simulink model "gm_sampleModel1912_4_sub"  (R2023a)
settings: Solver=VariableStepAuto  StartTime=0.0  StopTime=10.0  RelTol=1e-3
libraries: simulink x5
settings Model: Creator=user1  LastModifiedBy=user1
settings OptimizationCC: BlockReduction=off  ConditionallyExecuteInputs=off
settings DebuggingCC: InheritedTsInSrcMsg=none

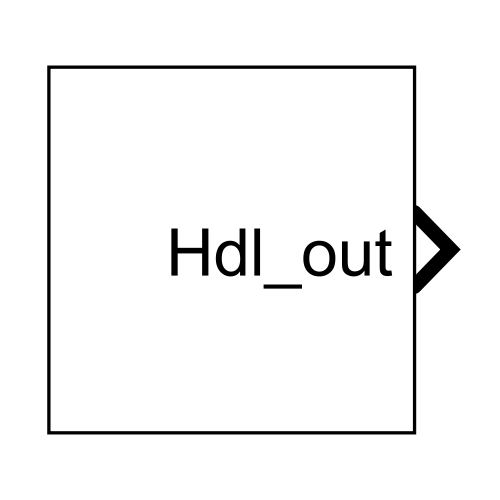
[thumbnail: Simulink's stored preview of the top-level diagram]
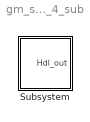
== system gm_sampleModel1912_4_sub ==
  Subsystem : Subsystem

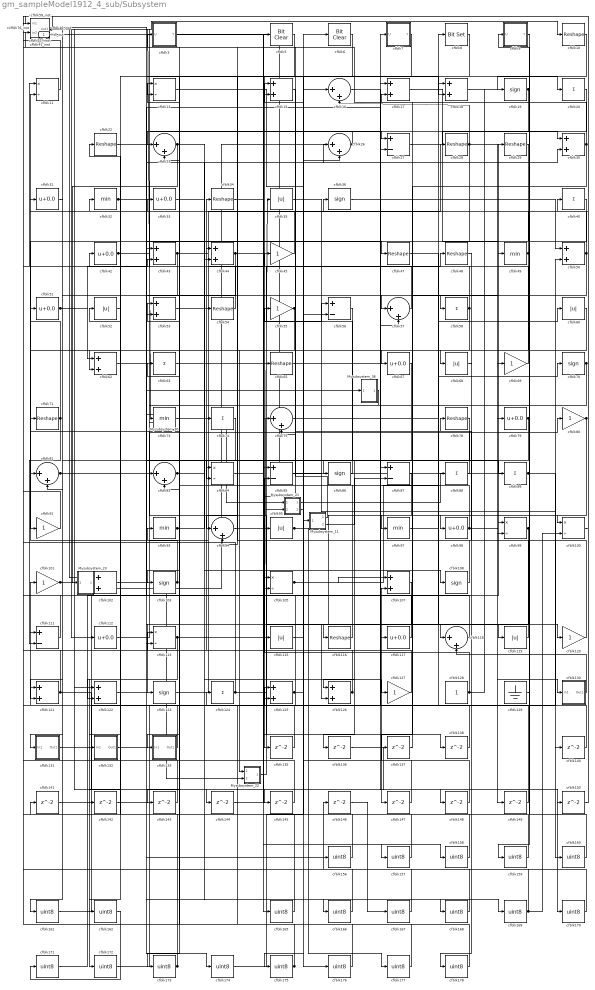
== system gm_sampleModel1912_4_sub/Subsystem ==
  Mysubsystem_11 : Subsystem
  Mysubsystem_21 : Subsystem
  Mysubsystem_22 : Subsystem
  Mysubsystem_23 : Subsystem
  Mysubsystem_30 : Subsystem
  Mysubsystem_36 : Subsystem
  cfblk{10,22,28..29,34,47..48,54,65,71,78,116} (12 alike) : Reshape
  cfblk{11,13,84,99..100,105,113} (7 alike) : Product  Inputs=*/  OutDataTypeStr=uint8  RndMeth=Zero  SaturateOnIntegerOverflow=on
  cfblk{45,55,69,80,91,101,120,127} (8 alike) : Gain  OutDataTypeStr=uint8
  cfblk{15,17..18,30,43..44,50,53,62,102,107,121..122,125..126} (15 alike) : Sum  OutDataTypeStr=uint8
  cfblk{19,36,70,86,103,108,123} (7 alike) : Signum
  cfblk106_inst : Subsystem
  cfblk{27,56,85,87,111} (5 alike) : Sum  Inputs=+-  OutDataTypeStr=uint8
  cfblk{31,33,42,51,67,79,98,112,117} (9 alike) : Bias  Bias=0.0  SaturateOnIntegerOverflow=off
  cfblk114_inst : Subsystem
  cfblk{35,52,60,68,95,115,119} (7 alike) : Abs  OutDataTypeStr=uint8  SaturateOnIntegerOverflow=off
  cfblk{16,23,26,57,75,81,83,94,118} (9 alike) : Sum  Inputs=|++  OutDataTypeStr=uint8
  cfblk{20,40,58,63,74,88..89,124} (8 alike) : Sum  Inputs=+  OutDataTypeStr=uint8
  cfblk128 : Constant  OutDataTypeStr=uint8  SampleTime=-1
  cfblk129 : Ground
  cfblk12_inst : Subsystem
  cfblk130 : Subsystem
  cfblk131 : Subsystem
  cfblk132 : Subsystem
  cfblk133 : Subsystem
  cfblk{135..138,140..150} (15 alike) : Delay  SampleTime=1
  cfblk14_inst : Subsystem
  cfblk{156..162,165..178} (21 alike) : DataTypeConversion  OutDataTypeStr=uint8  SaturateOnIntegerOverflow=off  RndMeth=Floor
  cfblk21_inst : Subsystem
  cfblk24_inst : Subsystem
  cfblk3 : Subsystem  mask(Detect Rise Positive){vinit=double(0), InputProcessing=Elements as channels (sample based), OutDataTypeStr=uint8}
      mask prompts: vinit "Simulink:masks:InitialCondition_MP"; InputProcessing "Simulink:masks:InputProcessing_MP"; OutDataTypeStr "Simulink:masks:OutputDataType_MP"
      mask help: Simulink:masks:DetectRisePositive_MD
      mask init:
      | InputProcessing = 'Elements as channels (sample based)';
      | OutDataTypeStr = 'uint8';
      | vinit = double(0);
      mask TypeOptions InputProcessing: Simulink:masks:ColumnsAsChannelsFrameBased | Simulink:masks:ElementsAsChannelsSampleBased
      mask TypeOptions OutDataTypeStr: Simulink:masks:uint8 | Simulink:masks:boolean
      mask Display: fprintf('U > 0\n&  NOT\nU/z > 0')
  cfblk{32,49,73,93,97} (5 alike) : MinMax  OutDataTypeStr=uint8
  cfblk37_inst : Subsystem
  cfblk38_inst : Subsystem
  cfblk4 : Constant  Value=0  OutDataTypeStr=uint8  SampleTime=1
  cfblk41_inst : Subsystem
  cfblk46_inst : Subsystem
  cfblk5 : simulink/Logic and Bit Operations/Bit Clear  iBit=0
      settings: LibrarySourceBlock=|
      | hdlsllib/Logic and Bit
      | Operations/Bit Clear
  cfblk59_inst : Subsystem
  cfblk6 : simulink/Logic and Bit Operations/Bit Clear  iBit=0
      settings: LibrarySourceBlock=|
      | hdlsllib/Logic and Bit
      | Operations/Bit Clear
  cfblk7 : Subsystem  mask(Detect Fall Nonpositive){vinit=double(0), InputProcessing=Elements as channels (sample based), OutDataTypeStr=uint8}
      mask prompts: vinit "Simulink:masks:InitialCondition_MP"; InputProcessing "Simulink:masks:InputProcessing_MP"; OutDataTypeStr "Simulink:masks:OutputDataType_MP"
      mask help: Simulink:masks:DetectFallNonpositive_MD
      mask init:
      | InputProcessing = 'Elements as channels (sample based)';
      | OutDataTypeStr = 'uint8';
      | vinit = double(0);
      mask TypeOptions InputProcessing: Simulink:masks:ColumnsAsChannelsFrameBased | Simulink:masks:ElementsAsChannelsSampleBased
      mask TypeOptions OutDataTypeStr: Simulink:masks:uint8 | Simulink:masks:boolean
      mask Display: fprintf('U <= 0\n&  NOT\nU/z <= 0')
  cfblk76_inst : Subsystem
  cfblk8 : simulink/Logic and Bit Operations/Bit Set  iBit=0
      settings: LibrarySourceBlock=|
      | hdlsllib/Logic and Bit
      | Operations/Bit Set
  cfblk9 : Subsystem  mask(Detect Fall Nonpositive){vinit=double(0), InputProcessing=Elements as channels (sample based), OutDataTypeStr=uint8}
      mask prompts: vinit "Simulink:masks:InitialCondition_MP"; InputProcessing "Simulink:masks:InputProcessing_MP"; OutDataTypeStr "Simulink:masks:OutputDataType_MP"
      mask help: Simulink:masks:DetectFallNonpositive_MD
      mask init:
      | InputProcessing = 'Elements as channels (sample based)';
      | OutDataTypeStr = 'uint8';
      | vinit = double(0);
      mask TypeOptions InputProcessing: Simulink:masks:ColumnsAsChannelsFrameBased | Simulink:masks:ElementsAsChannelsSampleBased
      mask TypeOptions OutDataTypeStr: Simulink:masks:uint8 | Simulink:masks:boolean
      mask Display: fprintf('U <= 0\n&  NOT\nU/z <= 0')
  cfblk92_inst : Subsystem
  Hdl_out : Outport  OutDataTypeStr=uint8  SampleTime=1
  wires:
  Mysubsystem_11/1(Out1) -> cfblk46_inst/2(in2)
  Mysubsystem_11/2(Out2) -> cfblk87/2
  Mysubsystem_21/1(Out1) -> cfblk88/1
  Mysubsystem_21/2(Out2) -> Mysubsystem_11/1(In1)
  Mysubsystem_22/1(Out1) -> Mysubsystem_21/2(In2)
  Mysubsystem_23/1(Out1) -> Mysubsystem_22/2(In2)
  Mysubsystem_30/1(Out1) -> Mysubsystem_21/1(In1)
  Mysubsystem_36/1(Out1) -> Mysubsystem_30/2(In2)
  cfblk10/1 -> cfblk135/1
  cfblk100/1 -> cfblk37_inst/1(in1)
  cfblk101/1 -> cfblk145/1, cfblk144/1
  cfblk102/1 -> cfblk80/1
  cfblk103/1 -> cfblk11/2, cfblk93/1
  cfblk105/1 -> cfblk18/1, cfblk107/1
  cfblk106_inst/1(out1) -> cfblk119/1
  cfblk107/1 -> cfblk123/1
  cfblk108/1 -> cfblk24_inst/1(in1)
  cfblk11/1 -> cfblk38_inst/1(in1)
  cfblk111/1 -> cfblk12_inst/1(in1)
  cfblk112/1 -> cfblk36/1
  cfblk113/1 -> cfblk35/1, cfblk172/1
  cfblk114_inst/1(out1) -> cfblk106_inst/1(in1), cfblk147/1
  cfblk115/1 -> cfblk56/2
  cfblk116/1 -> cfblk114_inst/1(in1)
  cfblk117/1 -> cfblk21_inst/1(in1)
  cfblk118/1 -> cfblk21_inst/2(in2)
  cfblk119/1 -> cfblk78/1
  cfblk12_inst/1(out1) -> cfblk27/1, cfblk73/1
  cfblk120/1 -> cfblk3/1(U)
  cfblk121/1 -> cfblk38_inst/2(in2), cfblk29/1, cfblk148/1
  cfblk122/1 -> cfblk174/1
  cfblk123/1 -> cfblk45/1
  cfblk124/1 -> cfblk48/1, cfblk37_inst/2(in2)
  cfblk125/1 -> cfblk26/2, cfblk16/1
  cfblk126/1 -> cfblk34/1, cfblk101/1
  cfblk127/1 -> cfblk52/1
  cfblk128/1 -> cfblk85/2, cfblk19/1
  cfblk129/1 -> cfblk49/1
  cfblk13/1 -> cfblk176/1
  cfblk130/1(Out1) -> cfblk118/2
  cfblk131/1(Out1) -> cfblk7/1(U)
  cfblk132/1(Out1) -> cfblk125/1
  cfblk133/1(Out1) -> cfblk111/1
  cfblk135/1 -> cfblk92_inst/1(in1)
  cfblk136/1 -> cfblk170/1
  cfblk137/1 -> cfblk17/2
  cfblk138/1 -> cfblk83/2
  cfblk14_inst/1(out1) -> cfblk85/1, cfblk122/1
  cfblk140/1 -> cfblk99/1
  cfblk141/1 -> cfblk50/2
  cfblk142/1 -> cfblk57/2
  cfblk143/1 -> cfblk59_inst/2(in2)
  cfblk144/1 -> cfblk56/1
  cfblk145/1 -> cfblk12_inst/2(in2)
  cfblk146/1 -> cfblk167/1
  cfblk147/1 -> cfblk15/1
  cfblk148/1 -> cfblk107/2
  cfblk149/1 -> cfblk105/1
  cfblk15/1 -> cfblk95/1
  cfblk150/1 -> cfblk40/1
  cfblk156/1 -> cfblk14_inst/2(in2)
  cfblk157/1 -> cfblk41_inst/1(in1)
  cfblk158/1 -> cfblk41_inst/2(in2)
  cfblk159/1 -> cfblk42/1
  cfblk16/1 -> cfblk87/1
  cfblk160/1 -> cfblk9/1(U)
  cfblk161/1 -> cfblk5/1
  cfblk162/1 -> cfblk171/1
  cfblk165/1 -> cfblk46_inst/1(in1)
  cfblk166/1 -> cfblk63/1
  cfblk167/1 -> cfblk76_inst/1(in1)
  cfblk168/1 -> cfblk146/1
  cfblk169/1 -> cfblk59_inst/1(in1), cfblk100/2
  cfblk17/1 -> cfblk69/1
  cfblk170/1 -> cfblk53/1
  cfblk171/1 -> cfblk53/2
  cfblk172/1 -> cfblk8/1
  cfblk173/1 -> cfblk106_inst/2(in2), cfblk141/1
  cfblk174/1 -> cfblk6/1
  cfblk175/1 -> cfblk113/1, cfblk124/1
  cfblk176/1 -> cfblk14_inst/1(in1)
  cfblk177/1 -> cfblk13/1
  cfblk178/1 -> cfblk13/2
  cfblk18/1 -> cfblk20/1
  cfblk19/1 -> cfblk27/2, cfblk23/2
  cfblk20/1 -> cfblk84/2
  cfblk21_inst/1(out1) -> cfblk18/2
  cfblk22/1 -> cfblk47/1
  cfblk23/1 -> cfblk54/1, Mysubsystem_23/1(In1)
  cfblk24_inst/1(out1) -> cfblk166/1
  cfblk26/1 -> cfblk23/1, cfblk102/2
  cfblk27/1 -> cfblk30/1
  cfblk28/1 -> cfblk79/1, cfblk75/2, cfblk16/2
  cfblk29/1 -> cfblk91/1
  cfblk3/1(Y) -> cfblk157/1
  cfblk30/1 -> cfblk24_inst/2(in2), cfblk137/1
  cfblk31/1 -> cfblk131/1(In1)
  cfblk32/1 -> cfblk149/1, cfblk74/1
  cfblk33/1 -> cfblk58/1
  cfblk34/1 -> cfblk168/1
  cfblk35/1 -> cfblk140/1
  cfblk36/1 -> cfblk50/1
  cfblk37_inst/1(out1) -> Mysubsystem_30/1(In1)
  cfblk38_inst/1(out1) -> cfblk102/1
  cfblk4/1 -> cfblk57/1
  cfblk40/1 -> cfblk67/1
  cfblk41_inst/1(out1) -> cfblk156/1
  cfblk42/1 -> cfblk83/1, cfblk75/1
  cfblk43/1 -> cfblk28/1, cfblk122/2
  cfblk44/1 -> cfblk62/2, cfblk161/1, cfblk158/1
  cfblk45/1 -> cfblk32/1
  cfblk46_inst/1(out1) -> cfblk86/1
  cfblk47/1 -> cfblk120/1
  cfblk48/1 -> cfblk118/1
  cfblk49/1 -> cfblk31/1, cfblk178/1
  cfblk5/1 -> cfblk162/1
  cfblk50/1 -> cfblk15/2, cfblk97/1
  cfblk51/1 -> cfblk62/1, cfblk43/2
  cfblk52/1 -> cfblk142/1
  cfblk53/1 -> cfblk169/1
  cfblk54/1 -> cfblk11/1
  cfblk55/1 -> cfblk94/2, cfblk143/1
  cfblk56/1 -> cfblk132/1(In1)
  cfblk57/1 -> cfblk22/1
  cfblk58/1 -> cfblk81/1, cfblk44/1, Mysubsystem_22/1(In1)
  cfblk59_inst/1(out1) -> cfblk112/1
  cfblk6/1 -> cfblk175/1
  cfblk60/1 -> cfblk68/1
  cfblk62/1 -> Mysubsystem_36/1(In1)
  cfblk63/1 -> cfblk165/1
  cfblk65/1 -> cfblk150/1
  cfblk67/1 -> cfblk103/1
  cfblk68/1 -> cfblk98/1
  cfblk69/1 -> cfblk92_inst/2(in2)
  cfblk7/1(Y) -> cfblk84/1
  cfblk70/1 -> cfblk99/2, cfblk105/2
  cfblk71/1 -> cfblk51/1, cfblk111/2
  cfblk73/1 -> cfblk115/1
  cfblk74/1 -> cfblk121/2
  cfblk75/1 -> cfblk70/1
  cfblk76_inst/1(out1) -> cfblk81/2, cfblk89/1
  cfblk78/1 -> cfblk94/1
  cfblk79/1 -> cfblk126/1, cfblk121/1, cfblk116/1
  cfblk8/1 -> cfblk173/1
  cfblk80/1 -> cfblk126/2, cfblk100/1
  cfblk81/1 -> cfblk26/1, cfblk17/1
  cfblk83/1 -> cfblk33/1, cfblk30/2, cfblk108/1
  cfblk84/1 -> cfblk138/1
  cfblk85/1 -> cfblk117/1
  cfblk86/1 -> cfblk55/1
  cfblk87/1 -> cfblk136/1
  cfblk88/1 -> cfblk76_inst/2(in2)
  cfblk89/1 -> cfblk160/1, Hdl_out/1
  cfblk9/1(Y) -> cfblk159/1
  cfblk91/1 -> cfblk114_inst/2(in2)
  cfblk92_inst/1(out1) -> cfblk44/2, cfblk10/1
  cfblk93/1 -> cfblk65/1, cfblk125/2
  cfblk94/1 -> cfblk127/1
  cfblk95/1 -> cfblk43/1, cfblk177/1
  cfblk97/1 -> cfblk60/1
  cfblk98/1 -> cfblk71/1, cfblk130/1(In1)
  cfblk99/1 -> cfblk113/2, cfblk133/1(In1)

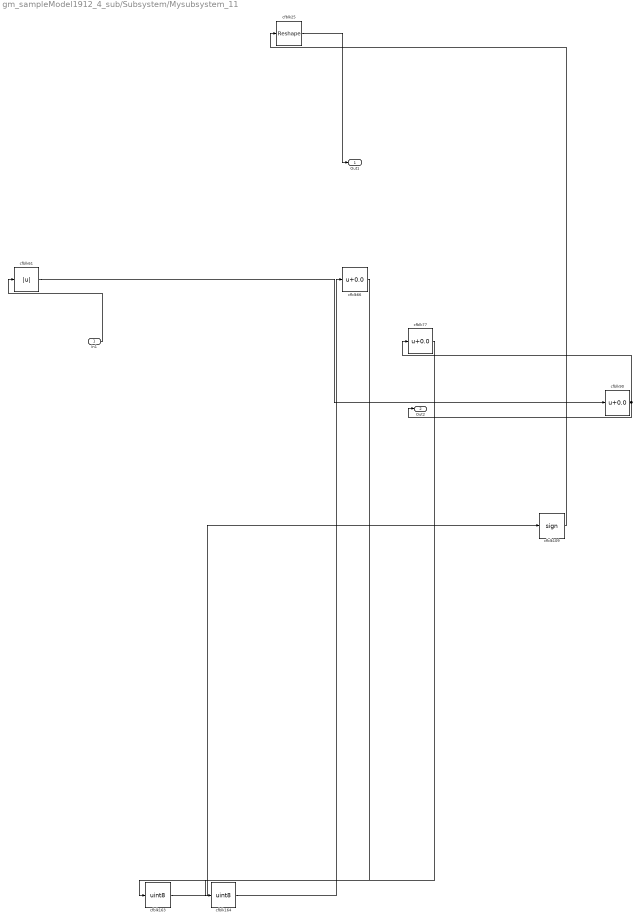
== system gm_sampleModel1912_4_sub/Subsystem/Mysubsystem_11 ==
  In1 : Inport  OutDataTypeStr=fixdt(0, 8, 7)  PortDimensions=1  SampleTime=1
  cfblk109 : Signum
  cfblk163 : DataTypeConversion  OutDataTypeStr=uint8  SaturateOnIntegerOverflow=off  RndMeth=Floor
  cfblk164 : DataTypeConversion  OutDataTypeStr=uint8  SaturateOnIntegerOverflow=off  RndMeth=Floor
  cfblk25 : Reshape
  cfblk61 : Abs  SaturateOnIntegerOverflow=off
  cfblk66 : Bias  Bias=0.0  SaturateOnIntegerOverflow=off
  cfblk77 : Bias  Bias=0.0  SaturateOnIntegerOverflow=off
  cfblk90 : Bias  Bias=0.0  SaturateOnIntegerOverflow=off
  Out1 : Outport  SampleTime=1
  Out2 : Outport  Port=2  SampleTime=1
  wires:
  In1/1 -> cfblk61/1
  cfblk109/1 -> cfblk25/1
  cfblk163/1 -> cfblk109/1
  cfblk164/1 -> cfblk66/1
  cfblk25/1 -> Out1/1
  cfblk61/1 -> cfblk90/1
  cfblk66/1 -> cfblk163/1
  cfblk77/1 -> cfblk164/1
  cfblk90/1 -> cfblk77/1, Out2/1

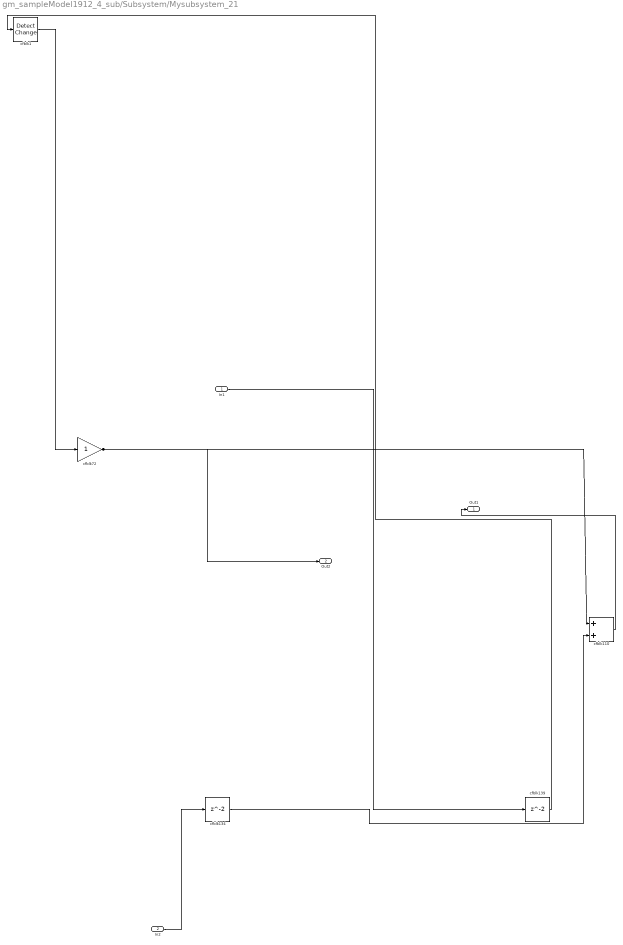
== system gm_sampleModel1912_4_sub/Subsystem/Mysubsystem_21 ==
  In1 : Inport  OutDataTypeStr=uint8  PortDimensions=1  SampleTime=1
  In2 : Inport  Port=2  OutDataTypeStr=uint8  PortDimensions=1  SampleTime=1
  cfblk1 : simulink/Logic and Bit Operations/Detect Change  vinit=0  OutDataTypeStr=boolean
      settings: LibrarySourceBlock=|
      | hdlsllib/Logic and Bit
      | Operations/Detect
      | Change
  cfblk110 : Sum
  cfblk134 : Delay  SampleTime=1
  cfblk139 : Delay  SampleTime=1
  cfblk72 : Gain
  Out1 : Outport  SampleTime=1
  Out2 : Outport  Port=2  SampleTime=1
  wires:
  In1/1 -> cfblk139/1
  In2/1 -> cfblk134/1
  cfblk1/1 -> cfblk72/1
  cfblk110/1 -> Out1/1
  cfblk134/1 -> cfblk110/2
  cfblk139/1 -> cfblk1/1
  cfblk72/1 -> cfblk110/1, Out2/1

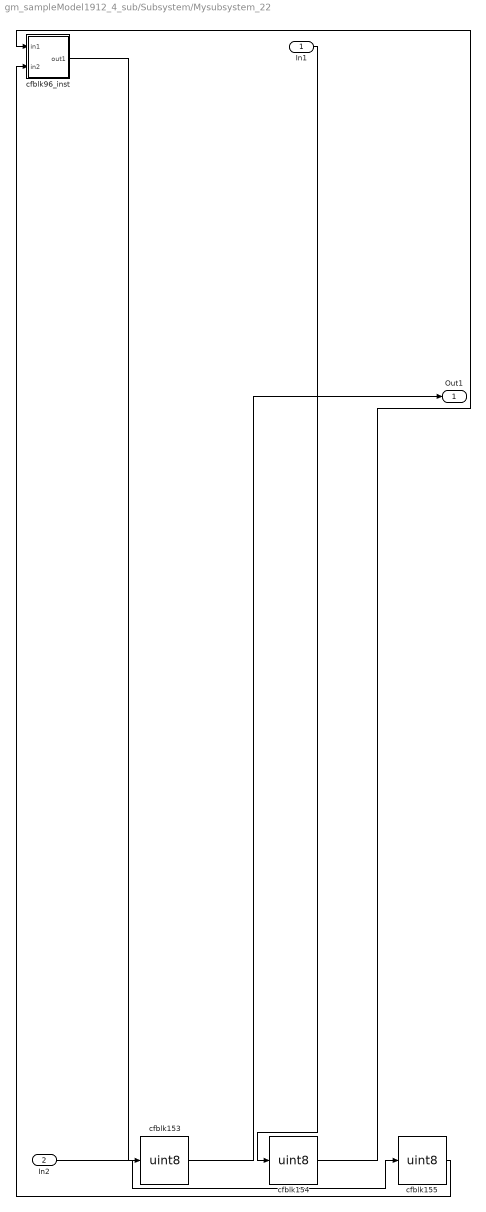
== system gm_sampleModel1912_4_sub/Subsystem/Mysubsystem_22 ==
  In1 : Inport  OutDataTypeStr=uint8  PortDimensions=1  SampleTime=1
  In2 : Inport  Port=2  OutDataTypeStr=uint8  PortDimensions=1  SampleTime=1
  cfblk153 : DataTypeConversion  OutDataTypeStr=uint8  SaturateOnIntegerOverflow=off  RndMeth=Floor
  cfblk154 : DataTypeConversion  OutDataTypeStr=uint8  SaturateOnIntegerOverflow=off  RndMeth=Floor
  cfblk155 : DataTypeConversion  OutDataTypeStr=uint8  SaturateOnIntegerOverflow=off  RndMeth=Floor
  cfblk96_inst : Subsystem
  Out1 : Outport  SampleTime=1
  wires:
  In1/1 -> cfblk154/1
  In2/1 -> cfblk155/1
  cfblk153/1 -> Out1/1
  cfblk154/1 -> cfblk96_inst/1(in1)
  cfblk155/1 -> cfblk96_inst/2(in2)
  cfblk96_inst/1(out1) -> cfblk153/1

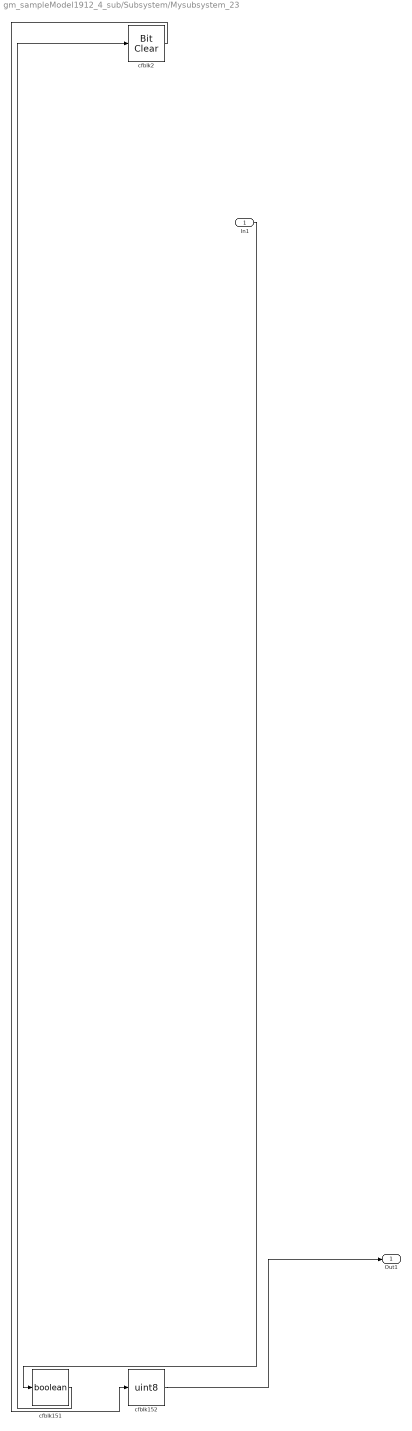
== system gm_sampleModel1912_4_sub/Subsystem/Mysubsystem_23 ==
  In1 : Inport  OutDataTypeStr=uint8  PortDimensions=1  SampleTime=1
  cfblk151 : DataTypeConversion  OutDataTypeStr=boolean  SaturateOnIntegerOverflow=off  RndMeth=Floor
  cfblk152 : DataTypeConversion  OutDataTypeStr=uint8  SaturateOnIntegerOverflow=off  RndMeth=Floor
  cfblk2 : simulink/Logic and Bit Operations/Bit Clear  iBit=0
      settings: LibrarySourceBlock=|
      | hdlsllib/Logic and Bit
      | Operations/Bit Clear
  Out1 : Outport  SampleTime=1
  wires:
  In1/1 -> cfblk151/1
  cfblk151/1 -> cfblk2/1
  cfblk152/1 -> Out1/1
  cfblk2/1 -> cfblk152/1

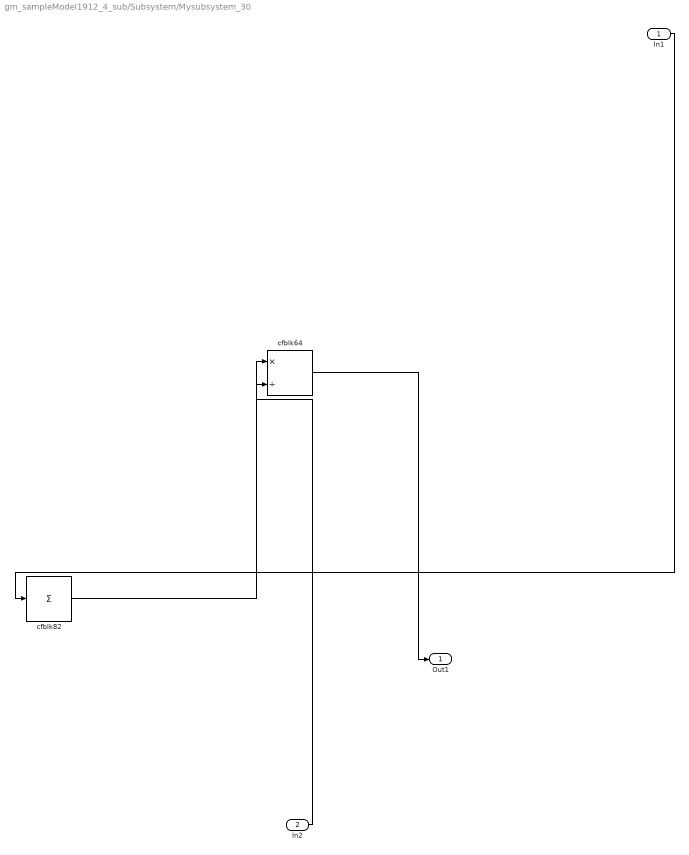
== system gm_sampleModel1912_4_sub/Subsystem/Mysubsystem_30 ==
  In1 : Inport  OutDataTypeStr=uint8  PortDimensions=1  SampleTime=1
  In2 : Inport  Port=2  OutDataTypeStr=uint8  PortDimensions=1  SampleTime=1
  cfblk64 : Product  Inputs=*/  RndMeth=Zero  SaturateOnIntegerOverflow=on
  cfblk82 : Sum  Inputs=+
  Out1 : Outport  SampleTime=1
  wires:
  In1/1 -> cfblk82/1
  In2/1 -> cfblk64/1
  cfblk64/1 -> Out1/1
  cfblk82/1 -> cfblk64/2

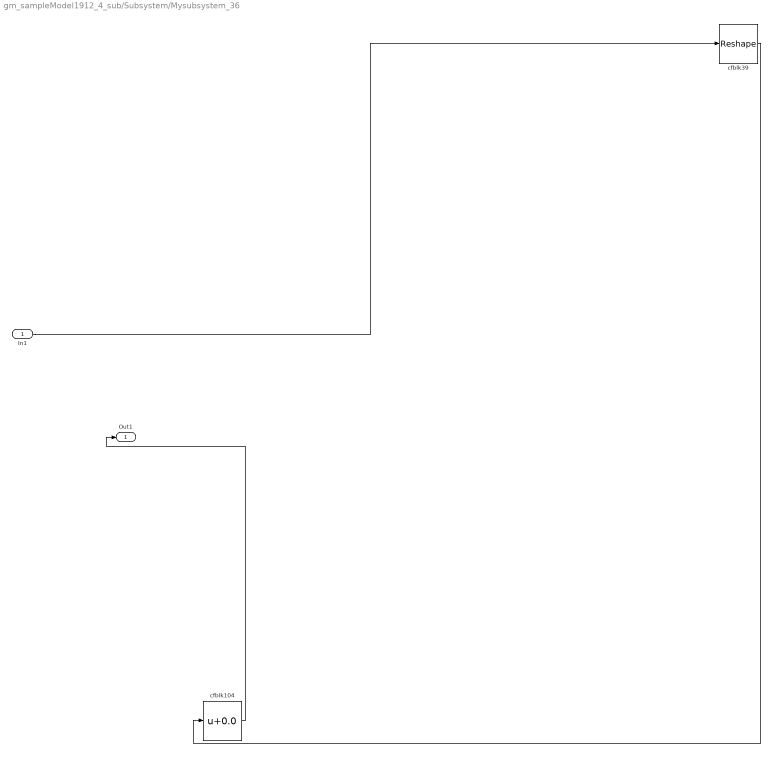
== system gm_sampleModel1912_4_sub/Subsystem/Mysubsystem_36 ==
  In1 : Inport  OutDataTypeStr=uint8  PortDimensions=1  SampleTime=1
  cfblk104 : Bias  Bias=0.0  SaturateOnIntegerOverflow=off
  cfblk39 : Reshape
  Out1 : Outport  SampleTime=1
  wires:
  In1/1 -> cfblk39/1
  cfblk104/1 -> Out1/1
  cfblk39/1 -> cfblk104/1

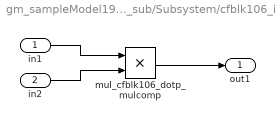
== system gm_sampleModel1912_4_sub/Subsystem/cfblk106_inst ==
  in1 : Inport  OutDataTypeStr=uint8  SampleTime=1
  in2 : Inport  Port=2  OutDataTypeStr=uint8  SampleTime=1
  mul_cfblk106_dotp_mulcomp : Product  Inputs=**  OutDataTypeStr=uint8  SampleTime=1
  out1 : Outport  OutDataTypeStr=uint8  SampleTime=1
  wires:
  in1/1 -> mul_cfblk106_dotp_mulcomp/1
  in2/1 -> mul_cfblk106_dotp_mulcomp/2
  mul_cfblk106_dotp_mulcomp/1 -> out1/1

== system gm_sampleModel1912_4_sub/Subsystem/cfblk114_inst ==
  in1 : Inport  OutDataTypeStr=uint8  SampleTime=1
  in2 : Inport  Port=2  OutDataTypeStr=uint8  SampleTime=1
  mul_cfblk114_dotp_mulcomp : Product  Inputs=**  OutDataTypeStr=uint8  SampleTime=1
  out1 : Outport  OutDataTypeStr=uint8  SampleTime=1
  wires:
  in1/1 -> mul_cfblk114_dotp_mulcomp/1
  in2/1 -> mul_cfblk114_dotp_mulcomp/2
  mul_cfblk114_dotp_mulcomp/1 -> out1/1

== system gm_sampleModel1912_4_sub/Subsystem/cfblk12_inst ==
  in1 : Inport  OutDataTypeStr=uint8  SampleTime=1
  in2 : Inport  Port=2  OutDataTypeStr=uint8  SampleTime=1
  mul_cfblk12_dotp_mulcomp : Product  Inputs=**  OutDataTypeStr=uint8  SampleTime=1
  out1 : Outport  OutDataTypeStr=uint8  SampleTime=1
  wires:
  in1/1 -> mul_cfblk12_dotp_mulcomp/1
  in2/1 -> mul_cfblk12_dotp_mulcomp/2
  mul_cfblk12_dotp_mulcomp/1 -> out1/1

== system gm_sampleModel1912_4_sub/Subsystem/cfblk130 ==
  In1 : Inport  OutDataTypeStr=uint8  PortDimensions=1  SampleTime=1
  Out1 : Outport  SampleTime=1
  wires:
  In1/1 -> Out1/1

== system gm_sampleModel1912_4_sub/Subsystem/cfblk131 ==
  In1 : Inport  OutDataTypeStr=uint8  PortDimensions=1  SampleTime=1
  Out1 : Outport  SampleTime=1
  wires:
  In1/1 -> Out1/1

== system gm_sampleModel1912_4_sub/Subsystem/cfblk132 ==
  In1 : Inport  OutDataTypeStr=uint8  PortDimensions=1  SampleTime=1
  Out1 : Outport  SampleTime=1
  wires:
  In1/1 -> Out1/1

== system gm_sampleModel1912_4_sub/Subsystem/cfblk133 ==
  In1 : Inport  OutDataTypeStr=uint8  PortDimensions=1  SampleTime=1
  Out1 : Outport  SampleTime=1
  wires:
  In1/1 -> Out1/1

== system gm_sampleModel1912_4_sub/Subsystem/cfblk14_inst ==
  in1 : Inport  OutDataTypeStr=uint8  SampleTime=1
  in2 : Inport  Port=2  OutDataTypeStr=uint8  SampleTime=1
  mul_cfblk14_dotp_mulcomp : Product  Inputs=**  OutDataTypeStr=uint8  SampleTime=1
  out1 : Outport  OutDataTypeStr=uint8  SampleTime=1
  wires:
  in1/1 -> mul_cfblk14_dotp_mulcomp/1
  in2/1 -> mul_cfblk14_dotp_mulcomp/2
  mul_cfblk14_dotp_mulcomp/1 -> out1/1

== system gm_sampleModel1912_4_sub/Subsystem/cfblk21_inst ==
  in1 : Inport  OutDataTypeStr=uint8  SampleTime=1
  in2 : Inport  Port=2  OutDataTypeStr=uint8  SampleTime=1
  mul_cfblk21_dotp_mulcomp : Product  Inputs=**  OutDataTypeStr=uint8  SampleTime=1
  out1 : Outport  OutDataTypeStr=uint8  SampleTime=1
  wires:
  in1/1 -> mul_cfblk21_dotp_mulcomp/1
  in2/1 -> mul_cfblk21_dotp_mulcomp/2
  mul_cfblk21_dotp_mulcomp/1 -> out1/1

== system gm_sampleModel1912_4_sub/Subsystem/cfblk24_inst ==
  in1 : Inport  OutDataTypeStr=uint8  SampleTime=1
  in2 : Inport  Port=2  OutDataTypeStr=uint8  SampleTime=1
  mul_cfblk24_dotp_mulcomp : Product  Inputs=**  OutDataTypeStr=uint8  SampleTime=1
  out1 : Outport  OutDataTypeStr=uint8  SampleTime=1
  wires:
  in1/1 -> mul_cfblk24_dotp_mulcomp/1
  in2/1 -> mul_cfblk24_dotp_mulcomp/2
  mul_cfblk24_dotp_mulcomp/1 -> out1/1

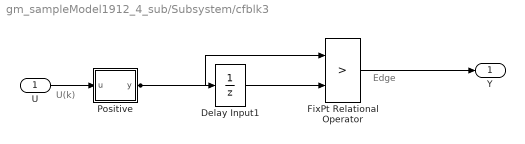
== system gm_sampleModel1912_4_sub/Subsystem/cfblk3 ==
  note: U(k)
  note: Edge
  U : Inport  OutDataTypeStr=uint8  SampleTime=1
  Delay Input1 : UnitDelay  Description=Store in Global RAM  DisableCoverage=on  InitialCondition=vinit  SampleTime=-1  HasFrameUpgradeWarning=on
  FixPt Relational Operator : RelationalOperator  Operator=>  OutDataTypeStr=fixdt(0, 8)  ZeroCross=off  InputSameDT=off
  Positive : Subsystem  mask(Compare To Zero){relop=>, OutDataTypeStr=boolean, ZeroCross=off}
      mask prompts: relop "Simulink:masks:Operator_MP"; OutDataTypeStr "Simulink:masks:OutputDataType_MP"; ZeroCross "Simulink:masks:EnableZerocrossingDetection_MP"
      mask help: Simulink:masks:CompareToZero_MD
      mask init:
      | OutDataTypeStr = 'boolean';
      | ZeroCross = 'off';
      | blkName = 'sampleModel1912_4_sub/Subsystem/cfblk3/Positive';
      | relop = '>';
      | setValue = 'boolean';
      mask TypeOptions relop: == | ~= | < | <= | >= | >
      mask TypeOptions OutDataTypeStr: Simulink:masks:uint8 | Simulink:masks:boolean
      mask Callback ZeroCross: sl('zeroCrossEnable', gcbh);
      mask Display: disp([relop,' 0'])
  Y : Outport  SampleTime=1
  wires:
  U/1 -> Positive/1(u)
  Delay Input1/1 -> FixPt Relational Operator/2
  FixPt Relational Operator/1 -> Y/1
  Positive/1(y) -> FixPt Relational Operator/1, Delay Input1/1

== system gm_sampleModel1912_4_sub/Subsystem/cfblk37_inst ==
  in1 : Inport  OutDataTypeStr=uint8  SampleTime=1
  in2 : Inport  Port=2  OutDataTypeStr=uint8  SampleTime=1
  mul_cfblk37_dotp_mulcomp : Product  Inputs=**  OutDataTypeStr=uint8  SampleTime=1
  out1 : Outport  OutDataTypeStr=uint8  SampleTime=1
  wires:
  in1/1 -> mul_cfblk37_dotp_mulcomp/1
  in2/1 -> mul_cfblk37_dotp_mulcomp/2
  mul_cfblk37_dotp_mulcomp/1 -> out1/1

== system gm_sampleModel1912_4_sub/Subsystem/cfblk38_inst ==
  in1 : Inport  OutDataTypeStr=uint8  SampleTime=1
  in2 : Inport  Port=2  OutDataTypeStr=uint8  SampleTime=1
  mul_cfblk38_dotp_mulcomp : Product  Inputs=**  OutDataTypeStr=uint8  SampleTime=1
  out1 : Outport  OutDataTypeStr=uint8  SampleTime=1
  wires:
  in1/1 -> mul_cfblk38_dotp_mulcomp/1
  in2/1 -> mul_cfblk38_dotp_mulcomp/2
  mul_cfblk38_dotp_mulcomp/1 -> out1/1

== system gm_sampleModel1912_4_sub/Subsystem/cfblk41_inst ==
  in1 : Inport  OutDataTypeStr=uint8  SampleTime=1
  in2 : Inport  Port=2  OutDataTypeStr=uint8  SampleTime=1
  mul_cfblk41_dotp_mulcomp : Product  Inputs=**  OutDataTypeStr=uint8  SampleTime=1
  out1 : Outport  OutDataTypeStr=uint8  SampleTime=1
  wires:
  in1/1 -> mul_cfblk41_dotp_mulcomp/1
  in2/1 -> mul_cfblk41_dotp_mulcomp/2
  mul_cfblk41_dotp_mulcomp/1 -> out1/1

== system gm_sampleModel1912_4_sub/Subsystem/cfblk46_inst ==
  in1 : Inport  OutDataTypeStr=uint8  SampleTime=1
  in2 : Inport  Port=2  OutDataTypeStr=uint8  SampleTime=1
  mul_cfblk46_dotp_mulcomp : Product  Inputs=**  OutDataTypeStr=uint8  SampleTime=1
  out1 : Outport  OutDataTypeStr=uint8  SampleTime=1
  wires:
  in1/1 -> mul_cfblk46_dotp_mulcomp/1
  in2/1 -> mul_cfblk46_dotp_mulcomp/2
  mul_cfblk46_dotp_mulcomp/1 -> out1/1

== system gm_sampleModel1912_4_sub/Subsystem/cfblk59_inst ==
  in1 : Inport  OutDataTypeStr=uint8  SampleTime=1
  in2 : Inport  Port=2  OutDataTypeStr=uint8  SampleTime=1
  mul_cfblk59_dotp_mulcomp : Product  Inputs=**  OutDataTypeStr=uint8  SampleTime=1
  out1 : Outport  OutDataTypeStr=uint8  SampleTime=1
  wires:
  in1/1 -> mul_cfblk59_dotp_mulcomp/1
  in2/1 -> mul_cfblk59_dotp_mulcomp/2
  mul_cfblk59_dotp_mulcomp/1 -> out1/1

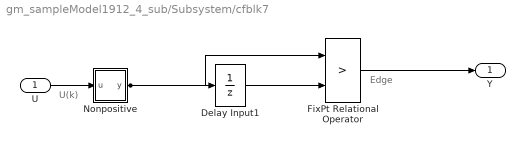
== system gm_sampleModel1912_4_sub/Subsystem/cfblk7 ==
  note: U(k)
  note: Edge
  U : Inport  OutDataTypeStr=uint8  SampleTime=1
  Delay Input1 : UnitDelay  Description=Store in Global RAM  DisableCoverage=on  InitialCondition=vinit  SampleTime=-1  HasFrameUpgradeWarning=on
  FixPt Relational Operator : RelationalOperator  Operator=>  OutDataTypeStr=fixdt(0, 8)  ZeroCross=off  InputSameDT=off
  Nonpositive : Subsystem  mask(Compare To Zero){relop=<=, OutDataTypeStr=boolean, ZeroCross=off}
      mask prompts: relop "Simulink:masks:Operator_MP"; OutDataTypeStr "Simulink:masks:OutputDataType_MP"; ZeroCross "Simulink:masks:EnableZerocrossingDetection_MP"
      mask help: Simulink:masks:CompareToZero_MD
      mask init:
      | OutDataTypeStr = 'boolean';
      | ZeroCross = 'off';
      | blkName = 'sampleModel1912_4_sub/Subsystem/cfblk7/Nonpositive';
      | relop = '<=';
      | setValue = 'boolean';
      mask TypeOptions relop: == | ~= | < | <= | >= | >
      mask TypeOptions OutDataTypeStr: Simulink:masks:uint8 | Simulink:masks:boolean
      mask Callback ZeroCross: sl('zeroCrossEnable', gcbh);
      mask Display: disp([relop,' 0'])
  Y : Outport  SampleTime=1
  wires:
  U/1 -> Nonpositive/1(u)
  Delay Input1/1 -> FixPt Relational Operator/2
  FixPt Relational Operator/1 -> Y/1
  Nonpositive/1(y) -> FixPt Relational Operator/1, Delay Input1/1

== system gm_sampleModel1912_4_sub/Subsystem/cfblk76_inst ==
  in1 : Inport  OutDataTypeStr=uint8  SampleTime=1
  in2 : Inport  Port=2  OutDataTypeStr=uint8  SampleTime=1
  mul_cfblk76_dotp_mulcomp : Product  Inputs=**  OutDataTypeStr=uint8  SampleTime=1
  out1 : Outport  OutDataTypeStr=uint8  SampleTime=1
  wires:
  in1/1 -> mul_cfblk76_dotp_mulcomp/1
  in2/1 -> mul_cfblk76_dotp_mulcomp/2
  mul_cfblk76_dotp_mulcomp/1 -> out1/1

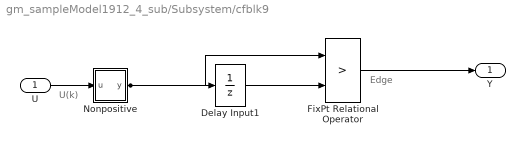
== system gm_sampleModel1912_4_sub/Subsystem/cfblk9 ==
  note: U(k)
  note: Edge
  U : Inport  OutDataTypeStr=uint8  SampleTime=1
  Delay Input1 : UnitDelay  Description=Store in Global RAM  DisableCoverage=on  InitialCondition=vinit  SampleTime=-1  HasFrameUpgradeWarning=on
  FixPt Relational Operator : RelationalOperator  Operator=>  OutDataTypeStr=fixdt(0, 8)  ZeroCross=off  InputSameDT=off
  Nonpositive : Subsystem  mask(Compare To Zero){relop=<=, OutDataTypeStr=boolean, ZeroCross=off}
      mask prompts: relop "Simulink:masks:Operator_MP"; OutDataTypeStr "Simulink:masks:OutputDataType_MP"; ZeroCross "Simulink:masks:EnableZerocrossingDetection_MP"
      mask help: Simulink:masks:CompareToZero_MD
      mask init:
      | OutDataTypeStr = 'boolean';
      | ZeroCross = 'off';
      | blkName = 'sampleModel1912_4_sub/Subsystem/cfblk9/Nonpositive';
      | relop = '<=';
      | setValue = 'boolean';
      mask TypeOptions relop: == | ~= | < | <= | >= | >
      mask TypeOptions OutDataTypeStr: Simulink:masks:uint8 | Simulink:masks:boolean
      mask Callback ZeroCross: sl('zeroCrossEnable', gcbh);
      mask Display: disp([relop,' 0'])
  Y : Outport  SampleTime=1
  wires:
  U/1 -> Nonpositive/1(u)
  Delay Input1/1 -> FixPt Relational Operator/2
  FixPt Relational Operator/1 -> Y/1
  Nonpositive/1(y) -> FixPt Relational Operator/1, Delay Input1/1

== system gm_sampleModel1912_4_sub/Subsystem/cfblk92_inst ==
  in1 : Inport  OutDataTypeStr=uint8  SampleTime=1
  in2 : Inport  Port=2  OutDataTypeStr=uint8  SampleTime=1
  mul_cfblk92_dotp_mulcomp : Product  Inputs=**  OutDataTypeStr=uint8  SampleTime=1
  out1 : Outport  OutDataTypeStr=uint8  SampleTime=1
  wires:
  in1/1 -> mul_cfblk92_dotp_mulcomp/1
  in2/1 -> mul_cfblk92_dotp_mulcomp/2
  mul_cfblk92_dotp_mulcomp/1 -> out1/1

== system gm_sampleModel1912_4_sub/Subsystem/Mysubsystem_22/cfblk96_inst ==
  in1 : Inport  OutDataTypeStr=uint8  SampleTime=1
  in2 : Inport  Port=2  OutDataTypeStr=uint8  SampleTime=1
  mul_cfblk96_dotp_mulcomp : Product  Inputs=**  OutDataTypeStr=uint16  SampleTime=1
  out1 : Outport  OutDataTypeStr=uint16  SampleTime=1
  wires:
  in1/1 -> mul_cfblk96_dotp_mulcomp/1
  in2/1 -> mul_cfblk96_dotp_mulcomp/2
  mul_cfblk96_dotp_mulcomp/1 -> out1/1

== system gm_sampleModel1912_4_sub/Subsystem/cfblk3/Positive ==
  u : Inport  OutDataTypeStr=uint8  SampleTime=1
  Compare : RelationalOperator  Operator=>  OutDataTypeStr=boolean  ZeroCross=off
  Constant : Constant  DisableCoverage=on  Value=0  OutDataTypeStr=Inherit: Inherit via back propagation  SampleTime=-1  PreserveConstantTs=on
  y : Outport  SampleTime=1
  wires:
  u/1 -> Compare/1
  Compare/1 -> y/1
  Constant/1 -> Compare/2

== system gm_sampleModel1912_4_sub/Subsystem/cfblk7/Nonpositive ==
  u : Inport  OutDataTypeStr=uint8  SampleTime=1
  Compare : RelationalOperator  Operator=<=  OutDataTypeStr=boolean  ZeroCross=off
  Constant : Constant  DisableCoverage=on  Value=0  OutDataTypeStr=Inherit: Inherit via back propagation  SampleTime=-1  PreserveConstantTs=on
  y : Outport  SampleTime=1
  wires:
  u/1 -> Compare/1
  Compare/1 -> y/1
  Constant/1 -> Compare/2

== system gm_sampleModel1912_4_sub/Subsystem/cfblk9/Nonpositive ==
  u : Inport  OutDataTypeStr=uint8  SampleTime=1
  Compare : RelationalOperator  Operator=<=  OutDataTypeStr=boolean  ZeroCross=off
  Constant : Constant  DisableCoverage=on  Value=0  OutDataTypeStr=Inherit: Inherit via back propagation  SampleTime=-1  PreserveConstantTs=on
  y : Outport  SampleTime=1
  wires:
  u/1 -> Compare/1
  Compare/1 -> y/1
  Constant/1 -> Compare/2
